simulink model "cint"  (Simulink 3.00)
settings: Solver=ode45  StartTime=0.0  StopTime=10.0  MaxStep=0.1  RelTol=1e-3  AbsTol=0.001
values from neighbouring files (symbols this model uses):
  A = real(a-J*c-b*K)    [css.m]    (also in lambor.m = [0 1 0 0)
  B = real(J)    [css.m]    (also in lambor.m = [0;16;0;0])
  C = real(K)    [css.m]    (also in lambor.m = [0 0 0 1])
  J = J'    [css.m]    (also in lambor.m)
  K = place(a,b,pc)    [css.m]    (also in paq.m = P*fii)
libraries: simulink3 x1
settings Model: TimeSaveName=t

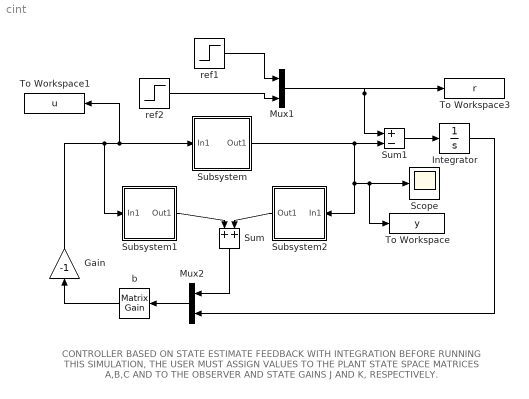
== system cint ==
  note: CONTROLLER BASED ON STATE ESTIMATE FEEDBACK WITH INTEGRATION
      | BEFORE RUNNING THIS SIMULATION,  THE USER MUST ASSIGN VALUES TO THE PLANT STATE SPACE
      | MATRICES A,B,C AND TO THE OBSERVER AND STATE GAINS J AND K, RESPECTIVELY.
  Gain : Gain  Orientation=up  Gain=-1  SaturateOnIntegerOverflow=on
  Integrator : Integrator  ExternalReset=none  InitialConditionSource=internal  InitialCondition=0  LimitOutput=off  UpperSaturationLimit=inf  LowerSaturationLimit=-inf  ShowSaturationPort=off  ShowStatePort=off  AbsoluteTolerance=auto
  Mux1 : Mux  Inputs=2
  Mux2 : Mux  Orientation=left  Inputs=2
  Scope : Scope
      settings: TimeRange=auto  YMin=-5  YMax=5  SaveToWorkspace=off  SaveName=ScopeData
  Subsystem : Subsystem  mask{A=A, B=B, C=C}
      mask Display: disp('PLANT')
  Subsystem1 : Subsystem  mask{A=A, B=B, C=C, J=J}
      mask init:
      | AT1=A-J*C; CT1=eye(size(A)); BT1=B;
      mask Display: disp('T_1')
  Subsystem2 : Subsystem  Orientation=left  mask{A=A, C=C, J=J}
      mask init:
      | AT2=A-J*C;BT2=J;CT2=eye(size(A));
      mask Display: disp('T_2')
  Sum : Sum  Orientation=down  Inputs=++  SaturateOnIntegerOverflow=off
  Sum1 : Sum  Inputs=+-  SaturateOnIntegerOverflow=off
  To Workspace : ToWorkspace  VariableName=y  SampleTime=-1  SaveFormat=Matrix
  To Workspace1 : ToWorkspace  VariableName=u  SampleTime=-1  SaveFormat=Matrix
  To Workspace3 : ToWorkspace  VariableName=r  SampleTime=-1  SaveFormat=Matrix
  b : simulink3/Math/Matrix Gain  Orientation=left  K=K
  ref1 : Step  Time=0  Before=0  After=1  SampleTime=0
  ref2 : Step  Time=5  Before=0  After=-1  SampleTime=0
  wires:
  Subsystem/1(Out1) -> Sum1/2, Scope/1, To Workspace/1, Subsystem2/1(In1)
  Subsystem1/1(Out1) -> Sum/1
  Subsystem2/1(Out1) -> Sum/2
  Sum1/1 -> Integrator/1
  Sum/1 -> Mux2/1
  Integrator/1 -> Mux2/2
  Mux2/1 -> b/1
  ref2/1 -> Mux1/2
  Mux1/1 -> Sum1/1, To Workspace3/1
  ref1/1 -> Mux1/1
  b/1 -> Gain/1
  Gain/1 -> Subsystem1/1(In1), Subsystem/1(In1), To Workspace1/1

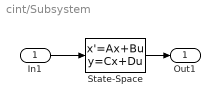
== system cint/Subsystem ==
  In1 : Inport  Port=1  PortWidth=-1  SampleTime=-1  DataType=auto
      settings: SignalType=auto
  State-Space : StateSpace  A=A  B=B  C=C  D=0*C*B  X0=0
  Out1 : Outport  Port=1
  wires:
  In1/1 -> State-Space/1
  State-Space/1 -> Out1/1

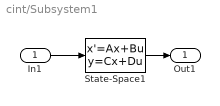
== system cint/Subsystem1 ==
  In1 : Inport  Port=1  PortWidth=-1  SampleTime=-1  DataType=auto
      settings: SignalType=auto
  State-Space1 : StateSpace  A=AT1  B=BT1  C=CT1  D=0*BT1  X0=0
  Out1 : Outport  Port=1
  wires:
  In1/1 -> State-Space1/1
  State-Space1/1 -> Out1/1

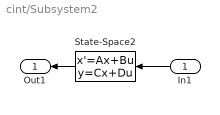
== system cint/Subsystem2 ==
  In1 : Inport  Orientation=left  Port=1  PortWidth=-1  SampleTime=-1  DataType=auto
      settings: SignalType=auto
  State-Space2 : StateSpace  Orientation=left  A=AT2  B=BT2  C=CT2  D=0* BT2  X0=0
  Out1 : Outport  Orientation=left  Port=1
  wires:
  In1/1 -> State-Space2/1
  State-Space2/1 -> Out1/1
